simulink model "hokuyo_ejemplo"  (Simulink 7.8)
settings: Solver=FixedStepDiscrete  StartTime=0.0  StopTime=inf  FixedStep=0.01  RelTol=1e-3
libraries: aerolibanimutils x1
settings Model: Creator=Sebastián  LastModifiedBy=Sebastián

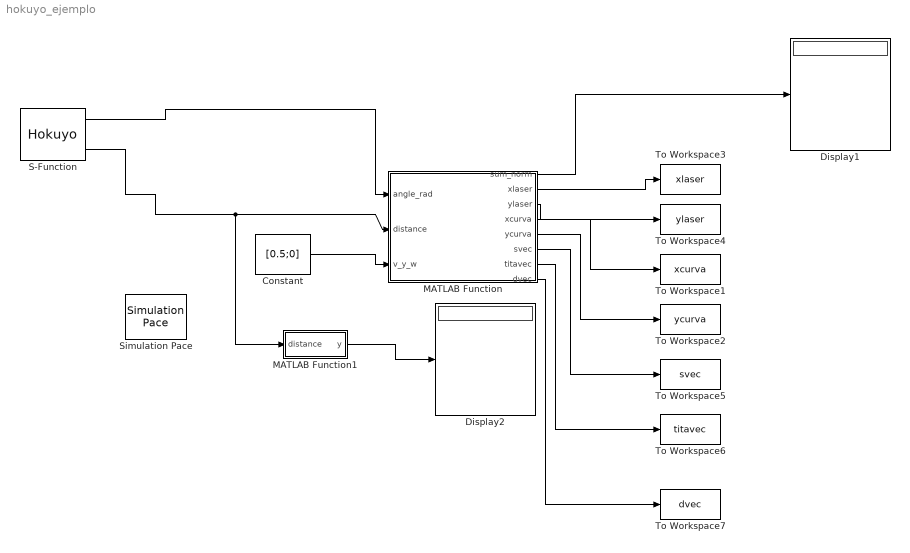
== system hokuyo_ejemplo ==
  Constant : Constant  Value=[0.5;0]
  Display1 : Display
  Display2 : Display
  MATLAB Function : MATLAB Function  TreatAsAtomicUnit=on
  MATLAB Function1 : MATLAB Function  TreatAsAtomicUnit=on
  S-Function : S-Function  FunctionName=Hokuyo  EnableBusSupport=off
  Simulation Pace : aerolibanimutils/Simulation Pace  SimulationPace=1  SleepMode=MATLAB Thread  OutputPaceError=off  SampleTime=-1
      settings: AttributesFormatString=%<SimulationPace> sec/sec
  To Workspace1 : ToWorkspace  VariableName=xcurva  SampleTime=-1  SaveFormat=Array
  To Workspace2 : ToWorkspace  VariableName=ycurva  SampleTime=-1  SaveFormat=Array
  To Workspace3 : ToWorkspace  VariableName=xlaser  SampleTime=-1  SaveFormat=Array
  To Workspace4 : ToWorkspace  VariableName=ylaser  SampleTime=-1  SaveFormat=Array
  To Workspace5 : ToWorkspace  VariableName=svec  SampleTime=-1  SaveFormat=Array
  To Workspace6 : ToWorkspace  VariableName=titavec  SampleTime=-1  SaveFormat=Array
  To Workspace7 : ToWorkspace  VariableName=dvec  SampleTime=-1  SaveFormat=Array
  wires:
  S-Function/1 -> MATLAB Function/1(angle_rad)
  S-Function/3 -> MATLAB Function/2(distance), MATLAB Function1/1(distance)
  Constant/1 -> MATLAB Function/3(v_y_w)
  MATLAB Function/1(sum_norm) -> Display1/1
  MATLAB Function1/1(y) -> Display2/1
  MATLAB Function/2(xlaser) -> To Workspace3/1
  MATLAB Function/3(ylaser) -> To Workspace4/1
  MATLAB Function/4(xcurva) -> To Workspace1/1
  MATLAB Function/5(ycurva) -> To Workspace2/1
  MATLAB Function/6(svec) -> To Workspace5/1
  MATLAB Function/7(titavec) -> To Workspace6/1
  MATLAB Function/8(dvec) -> To Workspace7/1

== matlab function MATLAB Function1 ==
  data: distance input double; y output double
function y = fcn(distance)
%#codegen

y=distance(342);

== matlab function MATLAB Function ==
  data: angle_rad input double; distance input double; sum_norm output double; v_y_w input double; xlaser output double; ylaser output double; xcurva output double; ycurva output double; svec output double; titavec output double; dvec output double
function [sum_norm,xlaser,ylaser,xcurva,ycurva,svec,titavec,dvec] = fcn(angle_rad,distance,v_y_w)
%#codegen

delta=0.3;
c=0.4;
s_max=1.5;
s_min=0.2;

if((abs(v_y_w(2))<0.0001))
    r=10000;
else
    r=abs(v_y_w(1))/abs(v_y_w(2));
end


if(v_y_w(2)>=0)
    xR=r;
else
    xR=-r;
end

xc=zeros(4,1);
yc=zeros(4,1);

sum=0;
p=0;

xlaser=zeros(683,1);
ylaser=zeros(683,1);

xcurva=zeros(683,1);
ycurva=zeros(683,1);

dvec=zeros(683,1);

svec=zeros(683,1);
titavec=zeros(683,1);

count=0;

for i=86:598
    
    if(distance(i)<4)
        xl=-distance(i)*sin(angle_rad(i))+xR;
        yl=distance(i)*cos(angle_rad(i));
        
        xlaser(i)=xl;
        ylaser(i)=yl;

        xc(1)=r*xl/sqrt(xl^2+yl^2);
        xc(2)=-r*xl/sqrt(xl^2+yl^2);
        xc(3)=r*xl/sqrt(xl^2+yl^2);
        xc(4)=-r*xl/sqrt(xl^2+yl^2);
        yc(1)=sqrt(r^2-xc(1)^2);
        yc(2)=sqrt(r^2-xc(2)^2);
        yc(3)=-sqrt(r^2-xc(3)^2);
        yc(4)=-sqrt(r^2-xc(4)^2);

        d=sqrt((xl-xc).^2+(yl-yc).^2);
        [d,j]=min(d);
        
        dvec(i)=d;
        
        xcurva(i)=xc(j);
        ycurva(i)=yc(j);
        
        tita=atan2(yc(j),xc(j));
        if(v_y_w(2)<0) 
            tita=pi-tita;
        end
        
        s=r*tita;
        
        svec(i)=s;
        titavec(i)=tita;
        
        if(s<s_max)
            
            if(d<=(c/2))
                p=1;
                count=count+1;
            end
            if((d>(c/2))&&(d<(delta+c/2)))
                  p=(1+cos((pi/delta)*(d-(c/2))))/2;
                  count=count+1;
            end
%             if(((c/2)<d)&&(d<(delta+c/2)))
%                 p=1-(d-c/2)/delta;
%                 count=count+1;
%             end
            if(d>=(delta+c/2))
                p=0;
            end
            
            if(s<s_min)
                s=s_min;
            end
            
            sum=sum+p*(s_max-s);
            
        end
        
    end
    
end

sum_norm=sum/((s_max-s_min)*513); %513 es la cantidad de lasers de -90 (laser 86) a 90 (laser 598) grado
sum_norm=sqrt(sum_norm);
